simulink library "rst"  (Simulink 8.1)
settings: Solver=ode1  StartTime=0.0  StopTime=Inf  FixedStep=0.001  RelTol=1e-3
PostLoadFcn:
  | , if any(exist('dsrtsu_mdlpostloadfcn', 'file') == [2, 3, 6]), try dsrtsu_mdlpostloadfcn('Execute', bdroot); catch fprintf('Error in PostLoadFcn (dsrtsu_mdlpostloadfcn) for model "%s":\n %s\n', bdroot, lasterr); end, end,
undefined symbols (not defined in the file or in its folder): FALSE, KACC_ACCGapErrorGParam_num, KACC_ACCGapFFParam_num, KACC_ACCGapInitialIParam_num, KACC_ACCGapKdParam_num, KACC_ACCGapKiParam_num, KACC_ACCGapMaxIParam_num, KACC_ACCGapMinIParam_num, KACC_ACCGapResetIParam_num
libraries: kpc x1, hcu_lib x1
settings Model: DSRTSU_INTERNAL_RTI_VER=450  DSRTSU_INTERNAL_RTI_TYPE=rti1401  RTICANMMDATA=struct('GeneralSetupData',struct('modelroot','D:\ELN150201_TAIWAN\trunk\AdasDragon\software\sw_development\arch\app\acc','generalsettings',struct('filesettings',struct('destfolder',struct('Name','RTICANMM_FILES','Check',1),'buildfolder',struct('Name','.','Check',1),'AbsDestfolder',struct('Name','D:\ELN150201_TAIWAN\trunk\AdasDragon\software\sw_development\arch\app\acc\RTICANMM_FILES'),'AbsBuildfolder',struct('Name','D:\ELN150201_TAIWAN\trunk\AdasDragon\software\sw_development\arch\app\acc'))),'options',struct('addpaths',1,'rmpaths',1,'addtrcexclusion',logical(1),'cannavigator',struct('checkmonitoring',0),'show_usrtrc',0,'use_usrtrc',0),'advanced',struct('options',[1 1 1 1 1 1 1 1 1 1 1 1 1 1 1 1 1 1 1 1 1 1 1 1 1 1 1 1 1 1 1 1 1 1 1 1 1 1 1 1 1 1 1 1 1 1 1 1 1 1 1 1 1 1 1 1 1 1 1 1 1 1 1 1 1 1 1 1 1 1 1 1 1 1 1 1 1 1 1 1 1 1 1 1 1 1 1 1 1 1 1 1 1 1 1 1 1 1 1 1]),'MPSetup',{{}},'modelname','rst','block','rst'))  DSRTSU_INTERNAL_RTIFPGA=40  Creator=AT015555  LastModifiedBy=AT015555

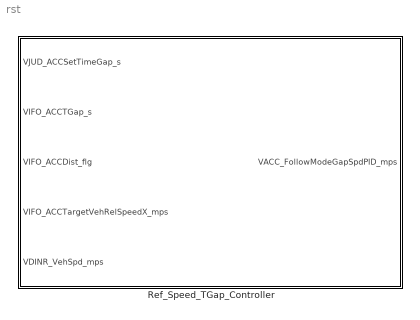
== system rst ==
  Ref_Speed_TGap_Controller : Subsystem

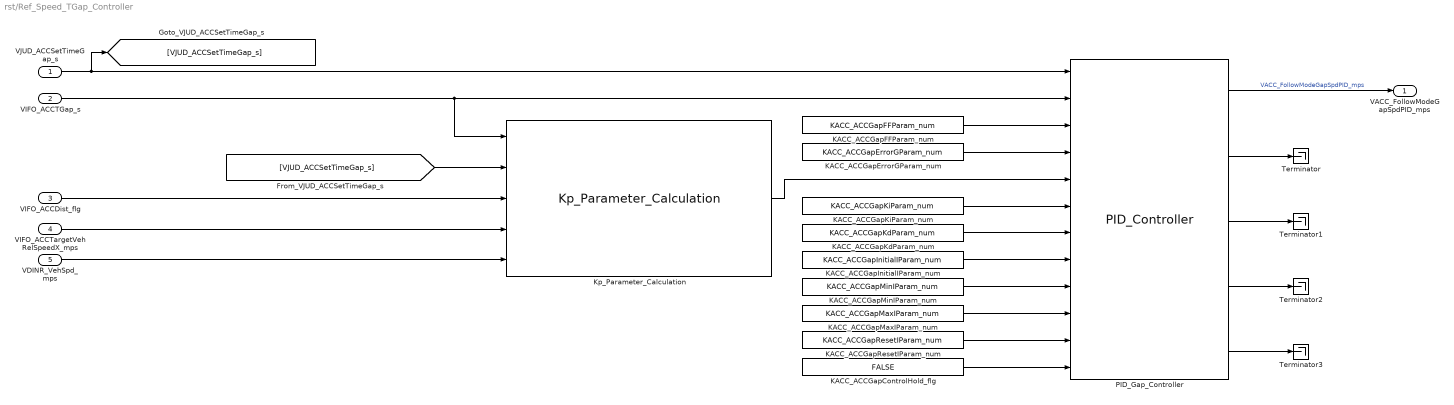
== system rst/Ref_Speed_TGap_Controller ==
  VJUD_ACCSetTimeGap_s : Inport
  VIFO_ACCTGap_s : Inport  Port=2
  VIFO_ACCDist_flg : Inport  Port=3
  VIFO_ACCTargetVehRelSpeedX_mps : Inport  Port=4
  VDINR_VehSpd_mps : Inport  Port=5
  KACC_ACCGapControlHold_flg : Constant  Value=FALSE  OutDataTypeStr=boolean
  KACC_ACCGapErrorGParam_num : Constant  Value=KACC_ACCGapErrorGParam_num
  KACC_ACCGapFFParam_num : Constant  Value=KACC_ACCGapFFParam_num
  KACC_ACCGapInitialIParam_num : Constant  Value=KACC_ACCGapInitialIParam_num
  KACC_ACCGapKdParam_num : Constant  Value=KACC_ACCGapKdParam_num
  KACC_ACCGapKiParam_num : Constant  Value=KACC_ACCGapKiParam_num
  KACC_ACCGapMaxIParam_num : Constant  Value=KACC_ACCGapMaxIParam_num
  KACC_ACCGapMinIParam_num : Constant  Value=KACC_ACCGapMinIParam_num
  KACC_ACCGapResetIParam_num : Constant  Value=KACC_ACCGapResetIParam_num
  Kp_Parameter_Calculation : kpc/Kp_Parameter_Calculation
  PID_Gap_Controller : hcu_lib/PID_Controller  SystemSampleTime=-1
  Terminator{,1..3} (4 alike) : Terminator
  VACC_FollowModeGapSpdPID_mps : Outport
  wires:
  KACC_ACCGapMaxIParam_num/1 -> PID_Gap_Controller/10
  KACC_ACCGapKiParam_num/1 -> PID_Gap_Controller/6
  Kp_Parameter_Calculation/1 -> PID_Gap_Controller/5
  VIFO_ACCTGap_s/1 -> Kp_Parameter_Calculation/1, PID_Gap_Controller/2
  PID_Gap_Controller/4 -> Terminator2/1
  PID_Gap_Controller/1 -> VACC_FollowModeGapSpdPID_mps/1  "VACC_FollowModeGapSpdPID_mps"
  PID_Gap_Controller/5 -> Terminator3/1
  KACC_ACCGapFFParam_num/1 -> PID_Gap_Controller/3
  VIFO_ACCDist_flg/1 -> Kp_Parameter_Calculation/3
  KACC_ACCGapInitialIParam_num/1 -> PID_Gap_Controller/8
  KACC_ACCGapErrorGParam_num/1 -> PID_Gap_Controller/4
  PID_Gap_Controller/2 -> Terminator/1
  PID_Gap_Controller/3 -> Terminator1/1
  KACC_ACCGapMinIParam_num/1 -> PID_Gap_Controller/9
  KACC_ACCGapKdParam_num/1 -> PID_Gap_Controller/7
  KACC_ACCGapResetIParam_num/1 -> PID_Gap_Controller/11
  [VJUD_ACCSetTimeGap_s] -> Kp_Parameter_Calculation/2
  VJUD_ACCSetTimeGap_s/1 -> [VJUD_ACCSetTimeGap_s], PID_Gap_Controller/1
  VIFO_ACCTargetVehRelSpeedX_mps/1 -> Kp_Parameter_Calculation/4
  KACC_ACCGapControlHold_flg/1 -> PID_Gap_Controller/12
  VDINR_VehSpd_mps/1 -> Kp_Parameter_Calculation/5
